simulink model "adder"  (R2016b)
settings: Solver=VariableStepAuto  StartTime=0.0  StopTime=10.0  RelTol=1e-3

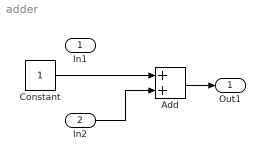
== system adder ==
  In1 : Inport
  In2 : Inport  Port=2
  Add : Sum
  Constant : Constant
  Out1 : Outport
  wires:
  Add/1 -> Out1/1
  In2/1 -> Add/2
  Constant/1 -> Add/1
